simulink model "Examen2_parte2"  (R2013a)
settings: Solver=ode23tb  StartTime=0.0  StopTime=10.0  RelTol=1e-3
libraries: powerlib x24
settings Model: Creator=Miguel  LastModifiedBy=Miguel

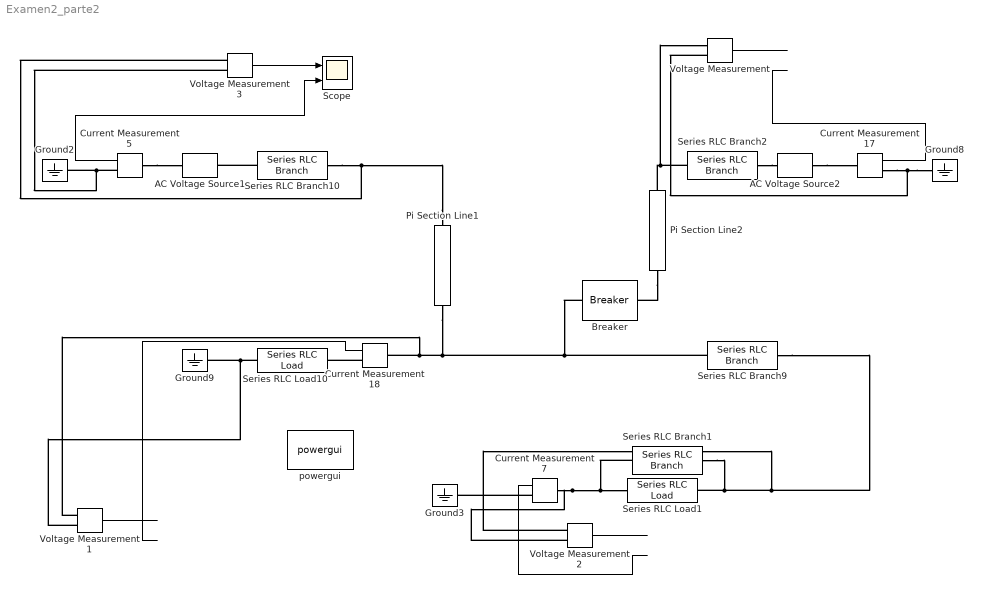
== system Examen2_parte2 ==
  AC Voltage Source1 : powerlib/Electrical Sources/AC Voltage Source  Amplitude=1.0*100e3*sqrt(2)  Phase=0  Frequency=60  SampleTime=0  Measurements=None
  AC Voltage Source2 : powerlib/Electrical Sources/AC Voltage Source  Amplitude=1.0*100e3*sqrt(2)  Phase=0.0712  Frequency=60  SampleTime=0  Measurements=None
  Breaker : powerlib/Elements/Breaker  BreakerResistance=0.001  InitialState=0  SnubberResistance=1e6  SnubberCapacitance=inf  SwitchingTimes=[ 1/60 ]  External=off  Measurements=None  MoreParameters=off  NoBreakLoop=off
  Current Measurement{5,7,17..18} (4 alike) : powerlib/Measurements/Current Measurement  PhasorSimulation=off  OutputType=Complex  PSBequivalent=0
  Ground{2..3,8..9} (4 alike) : powerlib/Elements/Ground  LConnTagsString=a
  Pi Section Line1 : powerlib/Elements/Pi Section Line  LConnTagsString=__new0  RConnTagsString=__new0  Frequency=60  Resistance=0.001*100e3^2/100e6  Inductance=0.05/(2*pi*60)*100e3^2/100e6  Capacitance=0.1/(2*pi*60*100e3^2/100e6)  Length=1  PiSections=1  Measurements=None
      settings: AttributesFormatString=\n
  Pi Section Line2 : powerlib/Elements/Pi Section Line  LConnTagsString=__new0  RConnTagsString=__new0  Frequency=60  Resistance=0.001*100e3^2/100e6  Inductance=0.05/(2*pi*60)*100e3^2/100e6  Capacitance=0.1/(2*pi*60*100e3^2/100e6)  Length=1  PiSections=1  Measurements=None
      settings: AttributesFormatString=\n
  Scope : Scope  NumInputPorts=2
      settings: ShowLegends=on  TimeRange=10  YMin=-5~-5  YMax=5~5
  Series RLC Branch1 : powerlib/Elements/Series RLC Branch  LConnTagsString=__new0  RConnTagsString=__new0  BranchType=C  Resistance=0  Inductance=0.1/(2*pi*60)*100e3^2/100e6  SetiL0=off  InitialCurrent=0  Capacitance=0.1/(2*pi*60*100e3^2/100e6)  Setx0=off  InitialVoltage=0  Measurements=None
  Series RLC Branch10 : powerlib/Elements/Series RLC Branch  LConnTagsString=__new0  RConnTagsString=__new0  BranchType=R  Resistance=1e-5  Inductance=1e-3  SetiL0=off  InitialCurrent=0  Capacitance=1e-6  Setx0=off  InitialVoltage=0  Measurements=None
  Series RLC Branch2 : powerlib/Elements/Series RLC Branch  LConnTagsString=__new0  RConnTagsString=__new0  BranchType=R  Resistance=1e-5  Inductance=1e-3  SetiL0=off  InitialCurrent=0  Capacitance=1e-6  Setx0=off  InitialVoltage=0  Measurements=None
  Series RLC Branch9 : powerlib/Elements/Series RLC Branch  LConnTagsString=__new0  RConnTagsString=__new0  BranchType=L  Resistance=0  Inductance=0.1/(2*pi*60)*100e3^2/100e6  SetiL0=off  InitialCurrent=0  Capacitance=1e-6  Setx0=off  InitialVoltage=0  Measurements=None
  Series RLC Load1 : powerlib/Elements/Series RLC Load  LConnTagsString=a  RConnTagsString=__new0  NominalVoltage=0.6922*100e3  NominalFrequency=60  ActivePower=100e6  InductivePower=100e6  CapacitivePower=0  Setx0=off  InitialVoltage=0  SetiL0=off  InitialCurrent=0  Measurements=Branch current
  Series RLC Load10 : powerlib/Elements/Series RLC Load  LConnTagsString=a  RConnTagsString=__new0  NominalVoltage=0.9264*100e3  NominalFrequency=60  ActivePower=100e6  InductivePower=100e6  CapacitivePower=0  Setx0=off  InitialVoltage=0  SetiL0=off  InitialCurrent=0  Measurements=Branch current
  Voltage Measurement{,1..3} (4 alike) : powerlib/Measurements/Voltage Measurement  PhasorSimulation=off  OutputType=Complex  PSBequivalent=0
  powergui : powerlib/powergui  Priority=1  SimulationMode=Continuous  SolverType=Tustin  SampleTime=50e-6  frequency=60  SPID=off  DisableSnubberDevices=off  DisableRonSwitches=off  DisableVfSwitches=off  SwTol=0  Interpol=off  DisplayEquations=off  frequencyindice=60  Pbase=100e6  ErrMax=1e-4  Iterations=50  UnitsV=kV  UnitsW=MW  FunctionMessages=off  echomessages=off  HookPort=off  EnableUseOfTLC=off  x0status=blocks  RestoreLinks=warning  ResistiveCurrentMeasurement=off  Frange=[0:2:500]  Ylog=off  Xlog=on  ShowGrid=off  save=off  variable=ZData  ZoomFFT=off  StartTime=0.0  cycles=1  DisplayStyle=1  fundamental=60  FreqAxis=off  MaxFrequency=1000  frequencyindicesteady=1  RmsSteady=2  display=off  Ts=0  methode=off
  wires:
  Voltage Measurement/1 -> ?
  Current Measurement17/1 -> ?
  Voltage Measurement1/1 -> ?
  Current Measurement18/1 -> ?
  Voltage Measurement2/1 -> ?
  Current Measurement7/1 -> ?
  Voltage Measurement3/1 -> Scope/1
  Current Measurement5/1 -> Scope/2
  connections:
  Current Measurement18/LConn1 -- Voltage Measurement1/LConn1 -- Breaker/LConn1 -- Series RLC Branch9/LConn1 -- Pi Section Line1/RConn1
  Pi Section Line1/LConn1 -- Series RLC Branch10/RConn1 -- Voltage Measurement3/LConn1
  Pi Section Line2/LConn1 -- Series RLC Branch2/RConn1 -- Voltage Measurement/LConn1
  Ground2/LConn1 -- Current Measurement5/RConn1 -- Voltage Measurement3/LConn2
  Voltage Measurement2/LConn2 -- Series RLC Branch1/LConn1 -- Series RLC Load1/LConn1 -- Current Measurement7/LConn1
  Voltage Measurement2/LConn1 -- Series RLC Branch1/RConn1 -- Series RLC Load1/RConn1 -- Series RLC Branch9/RConn1
  Ground8/LConn1 -- Current Measurement17/RConn1 -- Voltage Measurement/LConn2
  Ground9/LConn1 -- Series RLC Load10/LConn1 -- Voltage Measurement1/LConn2
  AC Voltage Source2/LConn1 -- Current Measurement17/LConn1
  Current Measurement7/RConn1 -- Ground3/LConn1
  Series RLC Branch10/LConn1 -- AC Voltage Source1/RConn1
  Series RLC Branch2/LConn1 -- AC Voltage Source2/RConn1
  Current Measurement5/LConn1 -- AC Voltage Source1/LConn1
  Current Measurement18/RConn1 -- Series RLC Load10/RConn1
  Pi Section Line2/RConn1 -- Breaker/RConn1
